simulink model "example_Hydraulic_AdditionalPump"  (R2016b)
settings: Solver=ode45  StartTime=0.0  StopTime=200  RelTol=1e-3  EnableMultiTasking=on
libraries: carnot x8, simulink x2
settings Model: Creator=drhf  LastModifiedBy=drhf
settings DataIOCC: LimitDataPoints=on  SaveFormat=Array  SignalLoggingSaveFormat=ModelDataLogs
settings OptimizationCC: ExpressionDepthLimit=2147483647  LifeSpan=inf
settings DebuggingCC: UnderspecifiedInitializationDetection=Classic  MergeDetectMultiDrivingBlocksExec=none  SolverPrmCheckMsg=warning  FcnCallInpInsideContextMsg=warning  StateNameClashWarn=warning  SFUnexpectedBacktrackingDiag=warning  SFNoUnconditionalDefaultTransitionDiag=warning  SFExecutionAtInitializationDiag=none
settings HardwareCC: ProdBitPerPointer=32  ProdBitPerSizeT=32  ProdBitPerPtrDiffT=32  ProdLargestAtomicFloat=None  ProdIntDivRoundTo=Undefined  ProdEndianess=Unspecified  ProdWordSize=32  ProdHWDeviceType=32-bit Generic
settings ModelReferenceCC: PropagateSignalLabelsOutOfModel=off
settings GRTTargetCC: TargetLangStandard=C89/C90 (ANSI)  GeneratePreprocessorConditionals=Disable all  CombineOutputUpdateFcns=off  GRTInterface=on
settings ConfigComp: CovMetricSettings=dw  CovHtmlReporting=on  CovSaveCumulativeToWorkspaceVar=on  CovSaveSingleToWorkspaceVar=on  CovExternalEMLEnable=off

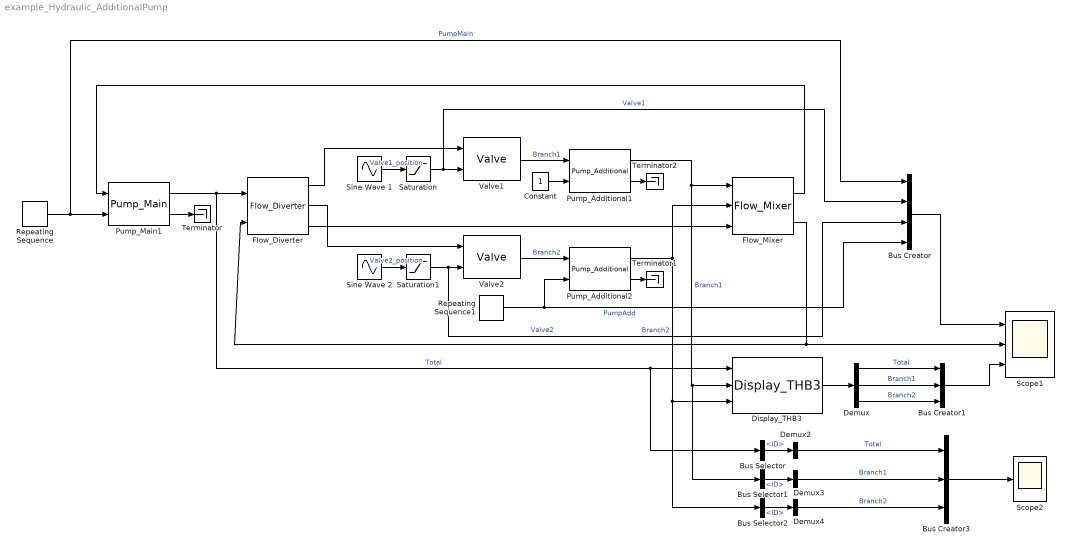
== system example_Hydraulic_AdditionalPump ==
  Bus Creator : BusCreator  Inputs=4
  Bus Creator1 : BusCreator  Inputs=3
  Bus Creator3 : BusCreator  Inputs=3
  Bus Selector : BusSelector  OutputSignals=ID
  Bus Selector1 : BusSelector  OutputSignals=ID
  Bus Selector2 : BusSelector  OutputSignals=ID
  Constant : Constant
  Demux : Demux  Outputs=3
  Demux2 : Demux  Outputs=1
  Demux3 : Demux  Outputs=1
  Demux4 : Demux  Outputs=1
  Display_THB3 : carnot/Outputs/Display_THB3  t=off  m=on  p=off  id=off  mix=off  d=off
  Flow_Diverter : carnot/Hydraulics/Flow_Diverter
  Flow_Mixer : carnot/Hydraulics/Flow_Mixer  t=1
  Pump_Additional1 : carnot/Hydraulics/Pump_Additional  a0=2.0e4  a1=-7000  a2=0 %-3e-3  dia=0.025  t1=1  ua=0  mcp=0  tamb=0
  Pump_Additional2 : carnot/Hydraulics/Pump_Additional  a0=2.0e4  a1=-7000  a2=0 %-3e-3  dia=0.025  t1=1  ua=0  mcp=0  tamb=0
  Pump_Main1 : carnot/Hydraulics/Pump_Main  a0=2.7e4  a1=-1.2e4  a2=0%-3e-3  dia=0.025  t1=5  p0=3e5  IDchk=off  fluid_id=Water  mix=0  ua=1  mcp=500  tamb=20
  Repeating Sequence : simulink/Sources/Repeating Sequence  rep_seq_t=[0 20 60 200]  rep_seq_y=[0 0 1 1]
  Repeating Sequence1 : simulink/Sources/Repeating Sequence  rep_seq_t="[0 80 100  200]"  rep_seq_y=[0 0 1 1]
  Saturation : Saturate  UpperLimit=1  LowerLimit=0
  Saturation1 : Saturate  UpperLimit=1  LowerLimit=0
  Scope1 : Scope  NumInputPorts=3
  Scope2 : Scope
  Sine Wave 1 : Sin  Amplitude=0.6  Bias=0.5  Frequency=1/20  SampleTime=0
  Sine Wave 2 : Sin  Amplitude=0.6  Bias=0.5  Frequency=1/20  Phase=pi  SampleTime=0
  Terminator : Terminator
  Terminator1 : Terminator
  Terminator2 : Terminator
  Valve1 : carnot/Hydraulics/Valve  pos_values=[0 0.1 1]  dp_values=[1e6 1e6 1]
  Valve2 : carnot/Hydraulics/Valve  pos_values=[0 0.1 1]  dp_values=[1e6 1e6 1]
  wires:
  Pump_Additional2/2 -> Terminator1/1
  Pump_Additional1/2 -> Terminator2/1
  Repeating Sequence/1 -> Pump_Main1/2, Bus Creator/1  "PumpMain"
  Pump_Main1/2 -> Terminator/1
  Sine Wave 1/1 -> Saturation/1  "Valve1_position"
  Flow_Diverter/1 -> Valve1/1
  Sine Wave 2/1 -> Saturation1/1  "Valve2_position"
  Flow_Diverter/2 -> Valve2/1
  Flow_Diverter/3 -> Flow_Mixer/3
  Flow_Mixer/2 -> Scope1/2, Flow_Diverter/2
  Flow_Mixer/1 -> Pump_Main1/1
  Bus Creator/1 -> Scope1/1
  Pump_Additional1/1 -> Bus Selector1/1, Display_THB3/2, Flow_Mixer/1  "Branch1"
  Pump_Additional2/1 -> Bus Selector2/1, Display_THB3/3, Flow_Mixer/2  "Branch2"
  Pump_Main1/1 -> Flow_Diverter/1, Bus Selector/1, Display_THB3/1  "Total"
  Display_THB3/1 -> Demux/1
  Demux/1 -> Bus Creator1/1  "Total"
  Demux/2 -> Bus Creator1/2  "Branch1"
  Demux/3 -> Bus Creator1/3  "Branch2"
  Bus Creator1/1 -> Scope1/3
  Saturation/1 -> Bus Creator/2, Valve1/2  "Valve1"
  Saturation1/1 -> Bus Creator/3, Valve2/2  "Valve2"
  Demux2/1 -> Bus Creator3/1  "Total"
  Demux4/1 -> Bus Creator3/3  "Branch2"
  Bus Creator3/1 -> Scope2/1
  Bus Selector/1 -> Demux2/1  "<ID>"
  Bus Selector1/1 -> Demux3/1  "<ID>"
  Demux3/1 -> Bus Creator3/2  "Branch1"
  Bus Selector2/1 -> Demux4/1  "<ID>"
  Valve1/1 -> Pump_Additional1/1  "Branch1"
  Constant/1 -> Pump_Additional1/2
  Valve2/1 -> Pump_Additional2/1  "Branch2"
  Repeating Sequence1/1 -> Bus Creator/4, Pump_Additional2/2  "PumpAdd"
